simulink model "deney5"  (R2023b)
settings: Solver=VariableStepAuto  StartTime=0.0  StopTime=10.0  RelTol=1e-3
libraries: commrandsrc3 x1
settings Model: Creator=fatih  LastModifiedBy=fatih

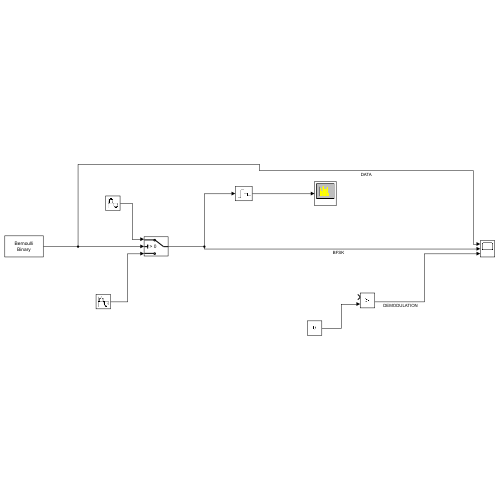
[thumbnail: Simulink's stored preview of the top-level diagram]
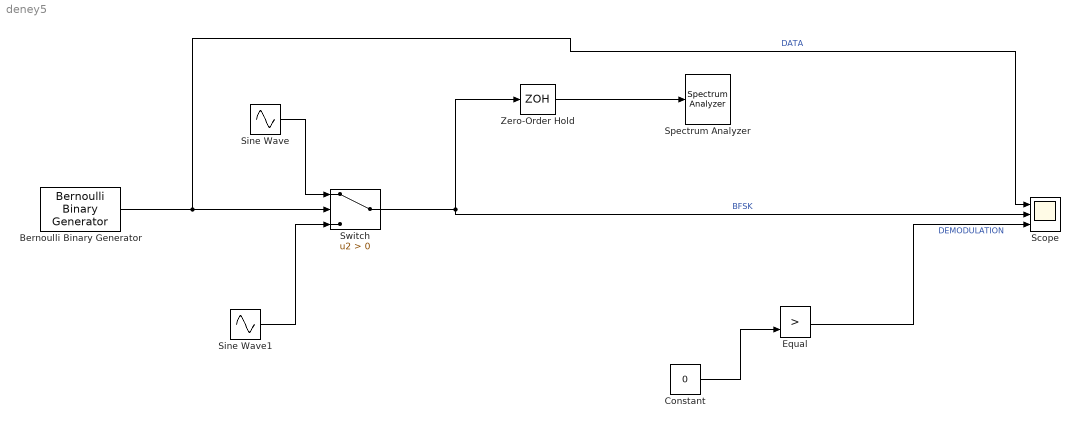
== system deney5 ==
  Bernoulli Binary Generator : commrandsrc3/Bernoulli Binary Generator  ProbabilityOfZero=0.5  SeedSource=Auto  Seed=0  SampleTime=1  SamplesPerFrame=1  OutputDataType=double  SimulateUsing=Interpreted execution
  Constant : Constant  Value=0
  Equal : RelationalOperator  Operator=>  OutDataTypeStr=boolean  RndMeth=Simplest  InputSameDT=off
  Scope : Scope  NumInputPorts=3
  Sine Wave : Sin  Frequency=18849.555921  SampleTime=0.00001
  Sine Wave1 : Sin  Frequency=6283.185307  SampleTime=0.00001
  Spectrum Analyzer : SpectrumAnalyzer  WindowPosition=[453.000000,230.000000,800.000000,500.000000,]  ScopeFrameLocation=window  Span=99999.99999999999  StartFrequency=-49999.99999999999  StopFrequency=49999.99999999999  YLimits=[-259.8120542,55.39753107]
  Switch : Switch  Criteria=u2 > Threshold  SaturateOnIntegerOverflow=off  InputSameDT=off
  Zero-Order Hold : ZeroOrderHold  SampleTime=0.00001
  wires:
  Zero-Order Hold/1 -> Spectrum Analyzer/1
  Bernoulli Binary Generator/1 -> Switch/2, Scope/1  "DATA"
  Switch/1 -> Zero-Order Hold/1, Scope/2  "BFSK"
  Equal/1 -> Scope/3  "DEMODULATION"
  Constant/1 -> Equal/2
  Sine Wave/1 -> Switch/1
  Sine Wave1/1 -> Switch/3
